simulink model "intensity_sim"  (R2020b)
settings: Solver=VariableStepAuto  StartTime=0.0  StopTime=stop_time  RelTol=1e-3
InitFcn:
  | intensity_sim_init
StopFcn:
  | intensity_sim_stop
values from neighbouring files (symbols this model uses):
  fs = 48000    [intensity_sim_init.m]
libraries: dspsrcs4 x5
settings Model: PacingRate=16  Creator=t96f346  LastModifiedBy=conno

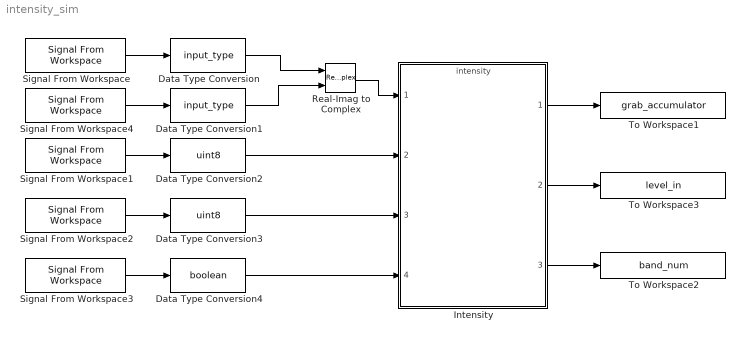
== system intensity_sim ==
  Data Type Conversion : DataTypeConversion  OutDataTypeStr=input_type
  Data Type Conversion1 : DataTypeConversion  OutDataTypeStr=input_type
  Data Type Conversion2 : DataTypeConversion  OutDataTypeStr=uint8
  Data Type Conversion3 : DataTypeConversion  OutDataTypeStr=uint8
  Data Type Conversion4 : DataTypeConversion  OutDataTypeStr=boolean
  Intensity : ModelReference  ModelNameDialog=intensity  SimulationMode=Normal  ModelReferenceVersion=2.35
  Real-Imag to Complex : RealImagToComplex
  Signal From Workspace : dspsrcs4/Signal From Workspace  X=FFT_data_real  Ts=1/fs  nsamps=1  OutputAfterFinalValue=Setting to zero  ignoreOrWarnInputAndFrameLengths=off  OutputFrames=off
  Signal From Workspace1 : dspsrcs4/Signal From Workspace  X=bin_num  Ts=1/fs  nsamps=1  OutputAfterFinalValue=Setting to zero  ignoreOrWarnInputAndFrameLengths=off  OutputFrames=off
  Signal From Workspace2 : dspsrcs4/Signal From Workspace  X=band_num  Ts=1/fs  nsamps=1  OutputAfterFinalValue=Setting to zero  ignoreOrWarnInputAndFrameLengths=off  OutputFrames=off
  Signal From Workspace3 : dspsrcs4/Signal From Workspace  X=valid_data  Ts=1/fs  nsamps=1  OutputAfterFinalValue=Setting to zero  ignoreOrWarnInputAndFrameLengths=off  OutputFrames=off
  Signal From Workspace4 : dspsrcs4/Signal From Workspace  X=FFT_data_imag  Ts=1/fs  nsamps=1  OutputAfterFinalValue=Setting to zero  ignoreOrWarnInputAndFrameLengths=off  OutputFrames=off
  To Workspace1 : ToWorkspace  VariableName=grab_accumulator  SampleTime=-1
      settings: Save2DSignal=2-D array (concatenate along first dimension)
  To Workspace2 : ToWorkspace  VariableName=band_num  SampleTime=-1
      settings: Save2DSignal=2-D array (concatenate along first dimension)
  To Workspace3 : ToWorkspace  VariableName=level_in  SampleTime=-1
      settings: Save2DSignal=2-D array (concatenate along first dimension)
  wires:
  Signal From Workspace/1 -> Data Type Conversion/1
  Signal From Workspace2/1 -> Data Type Conversion3/1
  Signal From Workspace3/1 -> Data Type Conversion4/1
  Intensity/3 -> To Workspace2/1
  Intensity/1 -> To Workspace1/1
  Intensity/2 -> To Workspace3/1
  Signal From Workspace1/1 -> Data Type Conversion2/1
  Real-Imag to Complex/1 -> Intensity/1
  Signal From Workspace4/1 -> Data Type Conversion1/1
  Data Type Conversion/1 -> Real-Imag to Complex/1
  Data Type Conversion1/1 -> Real-Imag to Complex/2
  Data Type Conversion2/1 -> Intensity/2
  Data Type Conversion3/1 -> Intensity/3
  Data Type Conversion4/1 -> Intensity/4
